simulink model "Part1A1"  (R2023a)
settings: Solver=VariableStepAuto  StartTime=0.0  StopTime=10.0  RelTol=1e-3
settings Model: Creator=rqouta  LastModifiedBy=rqouta

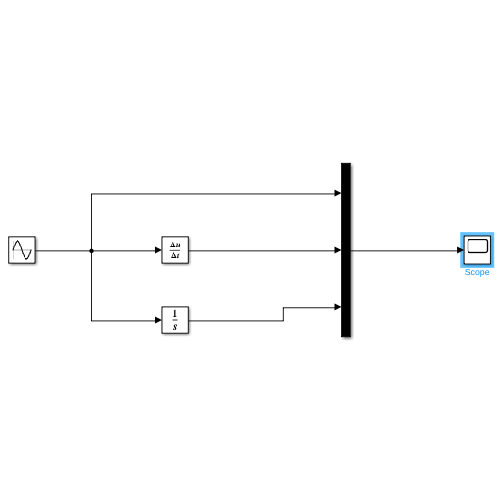
[thumbnail: Simulink's stored preview of the top-level diagram]
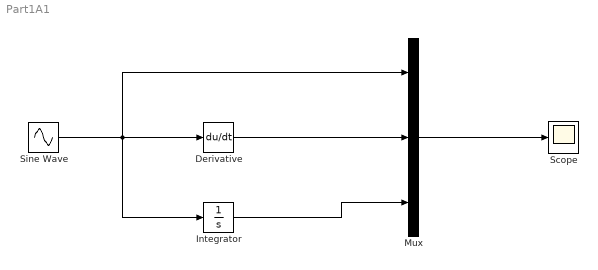
== system Part1A1 ==
  Derivative : Derivative
  Integrator : Integrator
  Mux : Mux  Inputs=3
  Scope : Scope
  Sine Wave : Sin  Frequency=1.256  SampleTime=0
  wires:
  Integrator/1 -> Mux/3
  Derivative/1 -> Mux/2
  Sine Wave/1 -> Mux/1, Integrator/1, Derivative/1
  Mux/1 -> Scope/1
